simulink model "gm_sampleModel1641_sub"  (R2023a)
settings: Solver=VariableStepAuto  StartTime=0.0  StopTime=10.0  RelTol=1e-3
libraries: hdlsllib x1, simulink x1
settings Model: Creator=user1  LastModifiedBy=user1
settings OptimizationCC: BlockReduction=off  ConditionallyExecuteInputs=off
settings DebuggingCC: InheritedTsInSrcMsg=none

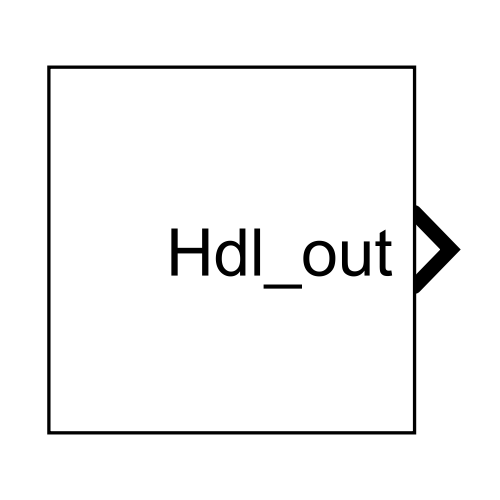
[thumbnail: Simulink's stored preview of the top-level diagram]
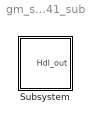
== system gm_sampleModel1641_sub ==
  Subsystem : Subsystem

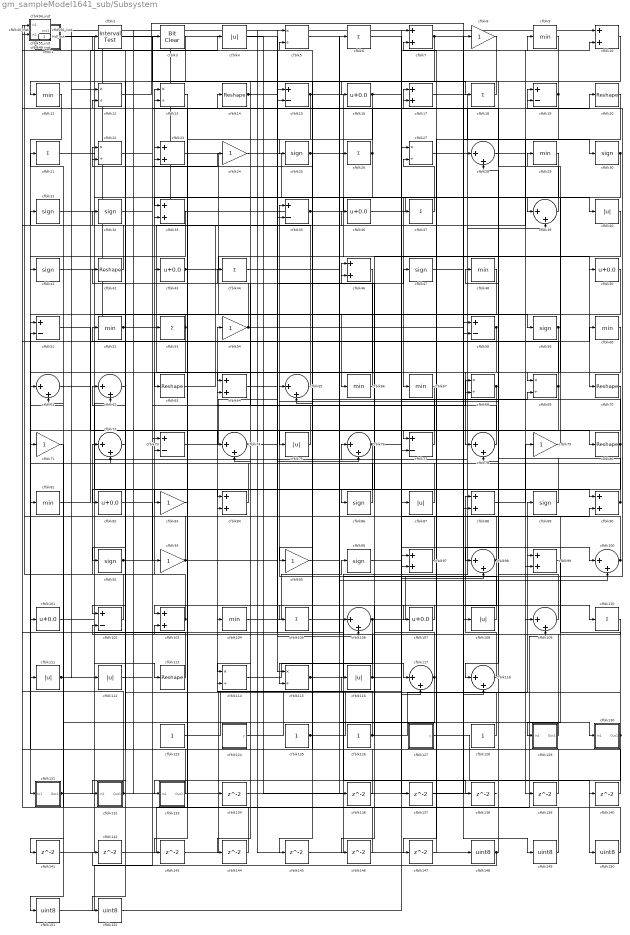
== system gm_sampleModel1641_sub/Subsystem ==
  cfblk1 : Subsystem  mask(Detect Fall Nonpositive){vinit=double(0), InputProcessing=Elements as channels (sample based), OutDataTypeStr=uint8}
      mask prompts: vinit "Simulink:masks:InitialCondition_MP"; InputProcessing "Simulink:masks:InputProcessing_MP"; OutDataTypeStr "Simulink:masks:OutputDataType_MP"
      mask help: Simulink:masks:DetectFallNonpositive_MD
      mask init:
      | InputProcessing = 'Elements as channels (sample based)';
      | OutDataTypeStr = 'uint8';
      | vinit = double(0);
      mask TypeOptions InputProcessing: Simulink:masks:ColumnsAsChannelsFrameBased | Simulink:masks:ElementsAsChannelsSampleBased
      mask TypeOptions OutDataTypeStr: Simulink:masks:uint8 | Simulink:masks:boolean
      mask Display: fprintf('U <= 0\n&  NOT\nU/z <= 0')
  cfblk{7,10,17,23,33,46,64,84,88,90,97,99,103} (13 alike) : Sum  OutDataTypeStr=uint8
  cfblk{28,39,61..62,65,72,74,76,78,98,100,106,109,117..118} (15 alike) : Sum  Inputs=|++  OutDataTypeStr=uint8
  cfblk{16,36,43,50,82,101,107} (7 alike) : Bias  Bias=0.0  SaturateOnIntegerOverflow=off
  cfblk{15,19,35,51,58,73,77,102} (8 alike) : Sum  Inputs=+-  OutDataTypeStr=uint8
  cfblk{9,11,29,48,52,60,66..67,81,104} (10 alike) : MinMax  OutDataTypeStr=uint8
  cfblk{6,18,21,26,37,44,53,105,110} (9 alike) : Sum  Inputs=+  OutDataTypeStr=uint8
  cfblk{4,40,75,87,108,111..112,116} (8 alike) : Abs  OutDataTypeStr=uint8  SaturateOnIntegerOverflow=off
  cfblk{14,20,42,63,70,80,113} (7 alike) : Reshape
  cfblk{5,12..13,22,27,68..69,114..115} (9 alike) : Product  Inputs=*/  OutDataTypeStr=uint8  RndMeth=Zero  SaturateOnIntegerOverflow=on
  cfblk{123,125..126,128} (4 alike) : Constant  OutDataTypeStr=uint8  SampleTime=-1
  cfblk124 : Subsystem  mask(Counter Free-Running){NumBits=double(16), tsamp=double(-1)}
      mask prompts: NumBits "Simulink:masks:NumberOfBits_MP"; tsamp "Simulink:masks:SampleTime_MP"
      mask help: Simulink:masks:CounterFreeRunning_MD
  cfblk127 : Subsystem  mask(Counter Limited){uplimit=double(7), tsamp=double(-1)}
      mask prompts: uplimit "Simulink:masks:UpperLimit_MP"; tsamp "Simulink:masks:SampleTime_MP"
      mask help: Simulink:masks:CounterLimited_MD
      mask init:
      | nbits = double(8);
      | tsamp = double(-1);
      | uplimit = double(7);
  cfblk129 : Subsystem
  cfblk130 : Subsystem
  cfblk131 : Subsystem
  cfblk132 : Subsystem
  cfblk133 : Subsystem
  cfblk{134,136..147} (13 alike) : Delay  SampleTime=1
  cfblk{148..152} (5 alike) : DataTypeConversion  OutDataTypeStr=uint8  SaturateOnIntegerOverflow=off  RndMeth=Floor
  cfblk2 : hdlsllib/Logic and Bit Operations/Interval Test  IntervalClosedRight=on  uplimit=0.5  IntervalClosedLeft=on  lowlimit=-0.5  OutDataTypeStr=uint8
  cfblk{8,24,54,71,79,83,93,95} (8 alike) : Gain  OutDataTypeStr=uint8
  cfblk{25,30..32,41,47,59,86,89,92,96} (11 alike) : Signum
  cfblk3 : simulink/Logic and Bit Operations/Bit Clear  iBit=0
      settings: LibrarySourceBlock=|
      | hdlsllib/Logic and Bit
      | Operations/Bit Clear
  cfblk34_inst : Subsystem
  cfblk45_inst : Subsystem
  cfblk49_inst : Subsystem
  cfblk55_inst : Subsystem
  cfblk56_inst : Subsystem
  cfblk94_inst : Subsystem
  Hdl_out : Outport  OutDataTypeStr=uint8  SampleTime=1
  wires:
  cfblk1/1(Y) -> cfblk90/1
  cfblk10/1 -> cfblk78/2
  cfblk100/1 -> cfblk34_inst/1(in1), cfblk13/1
  cfblk101/1 -> cfblk62/2
  cfblk102/1 -> cfblk94_inst/2(in2)
  cfblk103/1 -> cfblk73/2, cfblk72/1
  cfblk104/1 -> cfblk96/1
  cfblk105/1 -> cfblk138/1
  cfblk106/1 -> cfblk19/1, cfblk115/2
  cfblk107/1 -> cfblk103/1
  cfblk108/1 -> cfblk35/1
  cfblk109/1 -> cfblk65/1
  cfblk11/1 -> cfblk131/1(In1)
  cfblk110/1 -> cfblk103/2
  cfblk111/1 -> cfblk39/2, cfblk15/2, cfblk113/1
  cfblk112/1 -> cfblk76/1
  cfblk113/1 -> cfblk94_inst/1(in1)
  cfblk114/1 -> cfblk117/1
  cfblk115/1 -> cfblk19/2, cfblk5/2
  cfblk116/1 -> cfblk87/1, cfblk102/2, cfblk13/2, cfblk52/1
  cfblk117/1 -> cfblk46/1, cfblk151/1
  cfblk118/1 -> cfblk88/1
  cfblk12/1 -> cfblk58/1
  cfblk123/1 -> cfblk9/1
  cfblk124/1(y) -> cfblk116/1
  cfblk125/1 -> cfblk20/1, cfblk69/2
  cfblk126/1 -> cfblk89/1, cfblk46/2, cfblk54/1
  cfblk127/1(y) -> cfblk150/1
  cfblk128/1 -> cfblk62/1
  cfblk129/1(Out1) -> cfblk23/1
  cfblk13/1 -> cfblk63/1
  cfblk130/1(Out1) -> cfblk84/2, cfblk140/1, cfblk114/2, cfblk133/1(In1)
  cfblk131/1(Out1) -> cfblk99/1, cfblk6/1
  cfblk132/1(Out1) -> cfblk55_inst/2(in2), cfblk104/1
  cfblk133/1(Out1) -> cfblk22/1
  cfblk134/1 -> cfblk90/2
  cfblk136/1 -> cfblk56_inst/1(in1)
  cfblk137/1 -> cfblk28/1
  cfblk138/1 -> cfblk1/1(U)
  cfblk139/1 -> cfblk51/2
  cfblk14/1 -> cfblk106/2, cfblk114/1
  cfblk140/1 -> cfblk65/2
  cfblk141/1 -> cfblk5/1
  cfblk142/1 -> cfblk109/2
  cfblk143/1 -> cfblk27/1
  cfblk144/1 -> cfblk23/2
  cfblk145/1 -> cfblk98/2
  cfblk146/1 -> cfblk61/2
  cfblk147/1 -> cfblk7/2
  cfblk148/1 -> cfblk142/1, cfblk48/1
  cfblk149/1 -> cfblk49_inst/1(in1)
  cfblk15/1 -> cfblk70/1, cfblk33/1
  cfblk150/1 -> cfblk49_inst/2(in2)
  cfblk151/1 -> cfblk3/1
  cfblk152/1 -> cfblk97/2
  cfblk16/1 -> cfblk97/1, cfblk105/1
  cfblk17/1 -> cfblk139/1
  cfblk18/1 -> cfblk11/1
  cfblk19/1 -> cfblk77/1, cfblk16/1
  cfblk2/1 -> cfblk18/1
  cfblk20/1 -> cfblk118/1
  cfblk21/1 -> cfblk35/2
  cfblk22/1 -> cfblk17/1
  cfblk23/1 -> cfblk59/1
  cfblk24/1 -> cfblk67/1
  cfblk25/1 -> cfblk88/2, cfblk108/1
  cfblk26/1 -> cfblk64/1, cfblk45_inst/2(in2)
  cfblk27/1 -> cfblk30/1
  cfblk28/1 -> cfblk109/1
  cfblk29/1 -> cfblk107/1
  cfblk3/1 -> cfblk152/1
  cfblk30/1 -> cfblk69/1, cfblk143/1
  cfblk31/1 -> cfblk137/1
  cfblk32/1 -> cfblk17/2
  cfblk33/1 -> cfblk41/1
  cfblk34_inst/1(out1) -> cfblk134/1
  cfblk35/1 -> cfblk40/1, Hdl_out/1
  cfblk36/1 -> cfblk39/1
  cfblk37/1 -> cfblk27/2
  cfblk39/1 -> cfblk14/1
  cfblk4/1 -> cfblk37/1
  cfblk40/1 -> cfblk86/1
  cfblk41/1 -> cfblk106/1
  cfblk42/1 -> cfblk45_inst/1(in1)
  cfblk43/1 -> cfblk77/2, cfblk50/1
  cfblk44/1 -> cfblk136/1
  cfblk45_inst/1(out1) -> cfblk10/1
  cfblk46/1 -> cfblk75/1
  cfblk47/1 -> cfblk149/1
  cfblk48/1 -> cfblk66/1
  cfblk49_inst/1(out1) -> cfblk148/1
  cfblk5/1 -> cfblk130/1(In1)
  cfblk50/1 -> cfblk82/1
  cfblk51/1 -> cfblk80/1
  cfblk52/1 -> cfblk117/2, cfblk10/2, cfblk8/1
  cfblk53/1 -> cfblk51/1, cfblk111/1
  cfblk54/1 -> cfblk33/2, cfblk118/2, cfblk26/1
  cfblk55_inst/1(out1) -> cfblk12/1
  cfblk56_inst/1(out1) -> cfblk53/1
  cfblk58/1 -> cfblk78/1, cfblk74/2, cfblk102/1
  cfblk59/1 -> cfblk101/1, cfblk145/1
  cfblk6/1 -> cfblk99/2
  cfblk60/1 -> cfblk132/1(In1)
  cfblk61/1 -> cfblk4/1
  cfblk62/1 -> cfblk12/2
  cfblk63/1 -> cfblk36/1
  cfblk64/1 -> cfblk115/1
  cfblk65/1 -> cfblk56_inst/2(in2)
  cfblk66/1 -> cfblk42/1
  cfblk67/1 -> cfblk95/1
  cfblk68/1 -> cfblk83/1, cfblk81/1
  cfblk69/1 -> cfblk98/1, cfblk55_inst/1(in1)
  cfblk7/1 -> cfblk25/1, cfblk110/1
  cfblk70/1 -> cfblk147/1
  cfblk71/1 -> cfblk141/1
  cfblk72/1 -> cfblk32/1
  cfblk73/1 -> cfblk15/1
  cfblk74/1 -> cfblk76/2, cfblk144/1
  cfblk75/1 -> cfblk44/1
  cfblk76/1 -> cfblk84/1, cfblk100/1
  cfblk77/1 -> cfblk34_inst/2(in2)
  cfblk78/1 -> cfblk64/2
  cfblk79/1 -> cfblk29/1
  cfblk8/1 -> cfblk74/1
  cfblk80/1 -> cfblk92/1, cfblk22/2
  cfblk81/1 -> cfblk60/1
  cfblk82/1 -> cfblk93/1
  cfblk83/1 -> cfblk43/1
  cfblk84/1 -> cfblk71/1
  cfblk86/1 -> cfblk61/1
  cfblk87/1 -> cfblk72/2
  cfblk88/1 -> cfblk79/1
  cfblk89/1 -> cfblk68/1
  cfblk9/1 -> cfblk58/2
  cfblk90/1 -> cfblk73/1, cfblk28/2
  cfblk92/1 -> cfblk68/2, cfblk24/1
  cfblk93/1 -> cfblk47/1, cfblk21/1
  cfblk94_inst/1(out1) -> cfblk112/1
  cfblk95/1 -> cfblk100/2
  cfblk96/1 -> cfblk7/1
  cfblk97/1 -> cfblk31/1
  cfblk98/1 -> cfblk146/1, cfblk2/1
  cfblk99/1 -> cfblk129/1(In1)

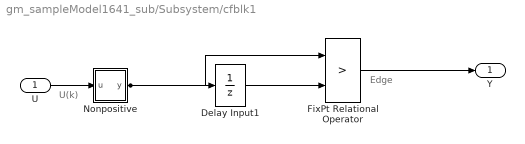
== system gm_sampleModel1641_sub/Subsystem/cfblk1 ==
  note: U(k)
  note: Edge
  U : Inport  OutDataTypeStr=uint8  SampleTime=1
  Delay Input1 : UnitDelay  Description=Store in Global RAM  DisableCoverage=on  InitialCondition=vinit  SampleTime=-1  HasFrameUpgradeWarning=on
  FixPt Relational Operator : RelationalOperator  Operator=>  OutDataTypeStr=fixdt(0, 8)  ZeroCross=off  InputSameDT=off
  Nonpositive : Subsystem  mask(Compare To Zero){relop=<=, OutDataTypeStr=boolean, ZeroCross=off}
      mask prompts: relop "Simulink:masks:Operator_MP"; OutDataTypeStr "Simulink:masks:OutputDataType_MP"; ZeroCross "Simulink:masks:EnableZerocrossingDetection_MP"
      mask help: Simulink:masks:CompareToZero_MD
      mask init:
      | OutDataTypeStr = 'boolean';
      | ZeroCross = 'off';
      | blkName = 'sampleModel1641_sub/Subsystem/cfblk1/Nonpositive';
      | relop = '<=';
      | setValue = 'boolean';
      mask TypeOptions relop: == | ~= | < | <= | >= | >
      mask TypeOptions OutDataTypeStr: Simulink:masks:uint8 | Simulink:masks:boolean
      mask Callback ZeroCross: sl('zeroCrossEnable', gcbh);
      mask Display: disp([relop,' 0'])
  Y : Outport  SampleTime=1
  wires:
  U/1 -> Nonpositive/1(u)
  Delay Input1/1 -> FixPt Relational Operator/2
  FixPt Relational Operator/1 -> Y/1
  Nonpositive/1(y) -> FixPt Relational Operator/1, Delay Input1/1

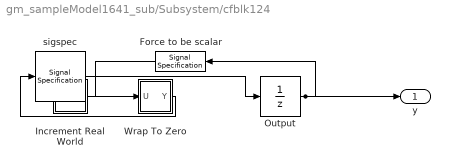
== system gm_sampleModel1641_sub/Subsystem/cfblk124 ==
  Force to be scalar : SignalSpecification  DisableCoverage=on  Dimensions=1
  Increment Real World : Subsystem  mask(Real World Value Increment){}
      mask help: Simulink:masks:RealWorldValueIncrement_MD
      mask Display: disp('V++')
  Output : UnitDelay  InitialCondition=0.0  SampleTime=tsamp  HasFrameUpgradeWarning=on
  Wrap To Zero : Subsystem  mask(Wrap To Zero){Threshold=double(65535)}
      mask prompts: Threshold "Simulink:masks:Threshold_MP"
      mask help: Simulink:masks:WrapToZero_MD
  sigspec : SignalSpecification  OutDataTypeStr=uint16  Dimensions=1
  y : Outport  SampleTime=1
  wires:
  Force to be scalar/1 -> Increment Real World/1(u)
  Increment Real World/1(y) -> Wrap To Zero/1(U)
  Output/1 -> Force to be scalar/1, y/1
  Wrap To Zero/1(Y) -> sigspec/1
  sigspec/1 -> Output/1

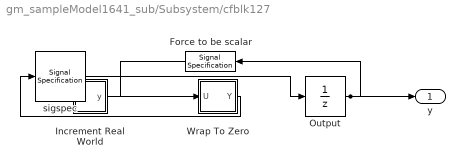
== system gm_sampleModel1641_sub/Subsystem/cfblk127 ==
  Force to be scalar : SignalSpecification  DisableCoverage=on  Dimensions=1
  Increment Real World : Subsystem  mask(Real World Value Increment){}
      mask help: Simulink:masks:RealWorldValueIncrement_MD
      mask Display: disp('V++')
  Output : UnitDelay  InitialCondition=0.0  SampleTime=tsamp  HasFrameUpgradeWarning=on
  Wrap To Zero : Subsystem  mask(Wrap To Zero){Threshold=double(7)}
      mask prompts: Threshold "Simulink:masks:Threshold_MP"
      mask help: Simulink:masks:WrapToZero_MD
  sigspec : SignalSpecification  OutDataTypeStr=uint8  Dimensions=1
  y : Outport  SampleTime=1
  wires:
  Force to be scalar/1 -> Increment Real World/1(u)
  Increment Real World/1(y) -> Wrap To Zero/1(U)
  Output/1 -> Force to be scalar/1, y/1
  Wrap To Zero/1(Y) -> sigspec/1
  sigspec/1 -> Output/1

== system gm_sampleModel1641_sub/Subsystem/cfblk129 ==
  In1 : Inport  OutDataTypeStr=uint8  PortDimensions=1  SampleTime=1
  Out1 : Outport  SampleTime=1
  wires:
  In1/1 -> Out1/1

== system gm_sampleModel1641_sub/Subsystem/cfblk130 ==
  In1 : Inport  OutDataTypeStr=uint8  PortDimensions=1  SampleTime=1
  Out1 : Outport  SampleTime=1
  wires:
  In1/1 -> Out1/1

== system gm_sampleModel1641_sub/Subsystem/cfblk131 ==
  In1 : Inport  OutDataTypeStr=uint8  PortDimensions=1  SampleTime=1
  Out1 : Outport  SampleTime=1
  wires:
  In1/1 -> Out1/1

== system gm_sampleModel1641_sub/Subsystem/cfblk132 ==
  In1 : Inport  OutDataTypeStr=uint8  PortDimensions=1  SampleTime=1
  Out1 : Outport  SampleTime=1
  wires:
  In1/1 -> Out1/1

== system gm_sampleModel1641_sub/Subsystem/cfblk133 ==
  In1 : Inport  OutDataTypeStr=uint8  PortDimensions=1  SampleTime=1
  Out1 : Outport  SampleTime=1
  wires:
  In1/1 -> Out1/1

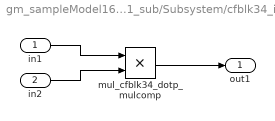
== system gm_sampleModel1641_sub/Subsystem/cfblk34_inst ==
  in1 : Inport  OutDataTypeStr=uint8  SampleTime=1
  in2 : Inport  Port=2  OutDataTypeStr=uint8  SampleTime=1
  mul_cfblk34_dotp_mulcomp : Product  Inputs=**  OutDataTypeStr=uint8  SampleTime=1
  out1 : Outport  OutDataTypeStr=uint8  SampleTime=1
  wires:
  in1/1 -> mul_cfblk34_dotp_mulcomp/1
  in2/1 -> mul_cfblk34_dotp_mulcomp/2
  mul_cfblk34_dotp_mulcomp/1 -> out1/1

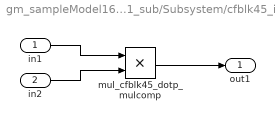
== system gm_sampleModel1641_sub/Subsystem/cfblk45_inst ==
  in1 : Inport  OutDataTypeStr=uint8  SampleTime=1
  in2 : Inport  Port=2  OutDataTypeStr=uint8  SampleTime=1
  mul_cfblk45_dotp_mulcomp : Product  Inputs=**  OutDataTypeStr=uint8  SampleTime=1
  out1 : Outport  OutDataTypeStr=uint8  SampleTime=1
  wires:
  in1/1 -> mul_cfblk45_dotp_mulcomp/1
  in2/1 -> mul_cfblk45_dotp_mulcomp/2
  mul_cfblk45_dotp_mulcomp/1 -> out1/1

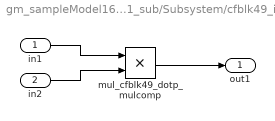
== system gm_sampleModel1641_sub/Subsystem/cfblk49_inst ==
  in1 : Inport  OutDataTypeStr=uint8  SampleTime=1
  in2 : Inport  Port=2  OutDataTypeStr=uint8  SampleTime=1
  mul_cfblk49_dotp_mulcomp : Product  Inputs=**  OutDataTypeStr=uint8  SampleTime=1
  out1 : Outport  OutDataTypeStr=uint8  SampleTime=1
  wires:
  in1/1 -> mul_cfblk49_dotp_mulcomp/1
  in2/1 -> mul_cfblk49_dotp_mulcomp/2
  mul_cfblk49_dotp_mulcomp/1 -> out1/1

== system gm_sampleModel1641_sub/Subsystem/cfblk55_inst ==
  in1 : Inport  OutDataTypeStr=uint8  SampleTime=1
  in2 : Inport  Port=2  OutDataTypeStr=uint8  SampleTime=1
  mul_cfblk55_dotp_mulcomp : Product  Inputs=**  OutDataTypeStr=uint8  SampleTime=1
  out1 : Outport  OutDataTypeStr=uint8  SampleTime=1
  wires:
  in1/1 -> mul_cfblk55_dotp_mulcomp/1
  in2/1 -> mul_cfblk55_dotp_mulcomp/2
  mul_cfblk55_dotp_mulcomp/1 -> out1/1

== system gm_sampleModel1641_sub/Subsystem/cfblk56_inst ==
  in1 : Inport  OutDataTypeStr=uint8  SampleTime=1
  in2 : Inport  Port=2  OutDataTypeStr=uint8  SampleTime=1
  mul_cfblk56_dotp_mulcomp : Product  Inputs=**  OutDataTypeStr=uint8  SampleTime=1
  out1 : Outport  OutDataTypeStr=uint8  SampleTime=1
  wires:
  in1/1 -> mul_cfblk56_dotp_mulcomp/1
  in2/1 -> mul_cfblk56_dotp_mulcomp/2
  mul_cfblk56_dotp_mulcomp/1 -> out1/1

== system gm_sampleModel1641_sub/Subsystem/cfblk94_inst ==
  in1 : Inport  OutDataTypeStr=uint8  SampleTime=1
  in2 : Inport  Port=2  OutDataTypeStr=uint8  SampleTime=1
  mul_cfblk94_dotp_mulcomp : Product  Inputs=**  OutDataTypeStr=uint8  SampleTime=1
  out1 : Outport  OutDataTypeStr=uint8  SampleTime=1
  wires:
  in1/1 -> mul_cfblk94_dotp_mulcomp/1
  in2/1 -> mul_cfblk94_dotp_mulcomp/2
  mul_cfblk94_dotp_mulcomp/1 -> out1/1

== system gm_sampleModel1641_sub/Subsystem/cfblk1/Nonpositive ==
  u : Inport  OutDataTypeStr=uint8  SampleTime=1
  Compare : RelationalOperator  Operator=<=  OutDataTypeStr=boolean  ZeroCross=off
  Constant : Constant  DisableCoverage=on  Value=0  OutDataTypeStr=Inherit: Inherit via back propagation  SampleTime=-1  PreserveConstantTs=on
  y : Outport  SampleTime=1
  wires:
  u/1 -> Compare/1
  Compare/1 -> y/1
  Constant/1 -> Compare/2

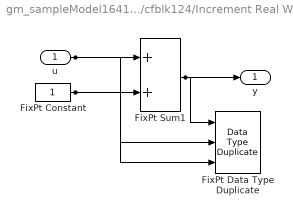
== system gm_sampleModel1641_sub/Subsystem/cfblk124/Increment Real World ==
  u : Inport  OutDataTypeStr=uint16  SampleTime=1
  FixPt Constant : Constant  DisableCoverage=on  OutDataTypeStr=Inherit: Inherit via back propagation  SampleTime=-1
  FixPt Data Type Duplicate : DataTypeDuplicate  DisableCoverage=on  NumInputPorts=3
  FixPt Sum1 : Sum  InputSameDT=on  OutDataTypeStr=Inherit: Inherit via back propagation  LockScale=on
  y : Outport  SampleTime=1
  wires:
  u/1 -> FixPt Sum1/1, FixPt Data Type Duplicate/2
  FixPt Constant/1 -> FixPt Sum1/2, FixPt Data Type Duplicate/3
  FixPt Sum1/1 -> FixPt Data Type Duplicate/1, y/1

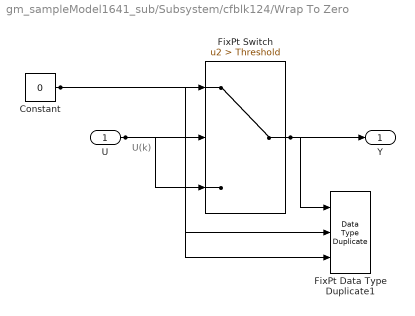
== system gm_sampleModel1641_sub/Subsystem/cfblk124/Wrap To Zero ==
  note: U(k)
  U : Inport  OutDataTypeStr=uint16  SampleTime=1
  Constant : Constant  DisableCoverage=on  Value=0  OutDataTypeStr=Inherit: Inherit via back propagation  SampleTime=-1
  FixPt Data Type Duplicate1 : DataTypeDuplicate  DisableCoverage=on  NumInputPorts=3
  FixPt Switch : Switch  Criteria=u2 > Threshold  Threshold=Threshold  OutDataTypeStr=Inherit: Inherit via back propagation  ZeroCross=off  SaturateOnIntegerOverflow=off  InputSameDT=off
  Y : Outport  SampleTime=1
  wires:
  U/1 -> FixPt Switch/3, FixPt Switch/2, FixPt Data Type Duplicate1/2
  Constant/1 -> FixPt Switch/1, FixPt Data Type Duplicate1/3
  FixPt Switch/1 -> FixPt Data Type Duplicate1/1, Y/1

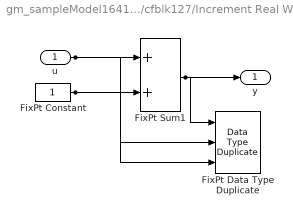
== system gm_sampleModel1641_sub/Subsystem/cfblk127/Increment Real World ==
  u : Inport  OutDataTypeStr=uint8  SampleTime=1
  FixPt Constant : Constant  DisableCoverage=on  OutDataTypeStr=Inherit: Inherit via back propagation  SampleTime=-1
  FixPt Data Type Duplicate : DataTypeDuplicate  DisableCoverage=on  NumInputPorts=3
  FixPt Sum1 : Sum  InputSameDT=on  OutDataTypeStr=Inherit: Inherit via back propagation  LockScale=on
  y : Outport  SampleTime=1
  wires:
  u/1 -> FixPt Sum1/1, FixPt Data Type Duplicate/2
  FixPt Constant/1 -> FixPt Sum1/2, FixPt Data Type Duplicate/3
  FixPt Sum1/1 -> FixPt Data Type Duplicate/1, y/1

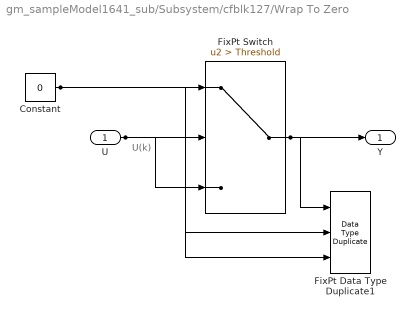
== system gm_sampleModel1641_sub/Subsystem/cfblk127/Wrap To Zero ==
  note: U(k)
  U : Inport  OutDataTypeStr=uint8  SampleTime=1
  Constant : Constant  DisableCoverage=on  Value=0  OutDataTypeStr=Inherit: Inherit via back propagation  SampleTime=-1
  FixPt Data Type Duplicate1 : DataTypeDuplicate  DisableCoverage=on  NumInputPorts=3
  FixPt Switch : Switch  Criteria=u2 > Threshold  Threshold=Threshold  OutDataTypeStr=Inherit: Inherit via back propagation  ZeroCross=off  SaturateOnIntegerOverflow=off  InputSameDT=off
  Y : Outport  SampleTime=1
  wires:
  U/1 -> FixPt Switch/3, FixPt Switch/2, FixPt Data Type Duplicate1/2
  Constant/1 -> FixPt Switch/1, FixPt Data Type Duplicate1/3
  FixPt Switch/1 -> FixPt Data Type Duplicate1/1, Y/1
